simulink model "Conditional_Integrated_Fuzzy_based_Sliding_Mode_Control"  (R2019a)
settings: Solver=FixedStepAuto  StartTime=0.0  StopTime=10  FixedStep=0.001  RelTol=1e-3  EnableMultiTasking=on
InitFcn:
  | %Variable_Entrada
  | Phi_max = 2000;
  | Phi_2  = 20;
  | Phi_1  = 1;
  | Phi_0  = 0;
  | %Variable_Salida
  | U_2= 0.218;
  | U_1 =0.16;
  | U_0  = 0;
  | 
  | %%
  | L =10;
  | Ki =1;
libraries: fuzblock x10
settings Model: Creator=alex_  LastModifiedBy=dell
settings DataIOCC: LimitDataPoints=on  SaveFormat=Array  ReturnWorkspaceOutputs=off
settings OptimizationCC: LifeSpan=inf
settings DebuggingCC: SolverPrmCheckMsg=warning  AllowSymbolicDim=off  SFUnexpectedBacktrackingDiag=warning  SFNoUnconditionalDefaultTransitionDiag=warning  SFExecutionAtInitializationDiag=none  ArithmeticOperatorsInVariantConditions=warning
settings HardwareCC: ProdBitPerPointer=32  ProdBitPerSizeT=32  ProdBitPerPtrDiffT=32  ProdLargestAtomicFloat=None  ProdIntDivRoundTo=Undefined  ProdEndianess=Unspecified  ProdWordSize=32  ProdHWDeviceType=32-bit Generic
settings ModelReferenceCC: PropagateSignalLabelsOutOfModel=off
settings SFSimCC: SimUseLocalCustomCode=off
settings RTWCC: RTWUseLocalCustomCode=off
settings CodeAppCC: StateflowObjectComments=on
settings GRTTargetCC: TargetLangStandard=C89/C90 (ANSI)  GeneratePreprocessorConditionals=Disable all
settings ConfigComp: CovMetricSettings=dw  CovHtmlReporting=on  CovSaveCumulativeToWorkspaceVar=on  CovSaveSingleToWorkspaceVar=on  CovExternalEMLEnable=off  CovSFcnEnable=off
settings SimscapeCC: SimscapeNormalizeSystem=off
settings ConfigurationSet: Description=SimMechanics 2G

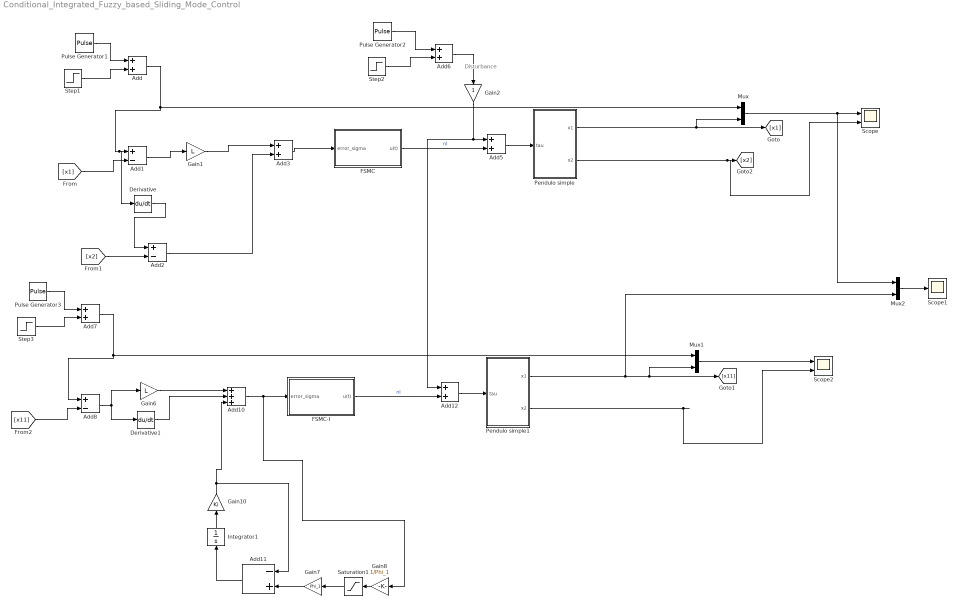
== system Conditional_Integrated_Fuzzy_based_Sliding_Mode_Control ==
  note: Disturbance
  Add{,3,5..7,12} (6 alike) : Sum
  Add1 : Sum  Inputs=+-
  Add10 : Sum  Inputs=+++
  Add11 : Sum  Inputs=-+
  Add2 : Sum  Inputs=+-
  Add8 : Sum  Inputs=+-
  Derivative : Derivative
  Derivative1 : Derivative
  "FSMC " : Subsystem
  FSMC-I : Subsystem
  Gain1 : Gain  Gain=L
  Gain10 : Gain  Gain=Ki
  Gain2 : Gain
  Gain6 : Gain  Gain=L
  Gain7 : Gain  Gain=Phi_1
  Gain8 : Gain  Gain=1/Phi_1
  Integrator1 : Integrator
  Mux : Mux  Inputs=2
  Mux1 : Mux  Inputs=2
  Mux2 : Mux  Inputs=2
  Pendulo simple : Subsystem
  Pendulo simple1 : Subsystem
  Pulse Generator1 : DiscretePulseGenerator  PulseType=Time based  Amplitude=-2  Period=5  PulseWidth=50
  Pulse Generator2 : DiscretePulseGenerator  PulseType=Time based  Amplitude=-0.32  Period=5  PulseWidth=50
  Pulse Generator3 : DiscretePulseGenerator  PulseType=Time based  Amplitude=-2  Period=5  PulseWidth=50
  Saturation1 : Saturate  UpperLimit=1  LowerLimit=-1
  Scope : Scope  NumInputPorts=2
  Scope1 : Scope
  Scope2 : Scope  NumInputPorts=2
  Step1 : Step  Time=0  SampleTime=0
  Step2 : Step  Time=0  After=0.16  SampleTime=0
  Step3 : Step  Time=0  SampleTime=0
  wires:
  Mux/1 -> Mux2/1, Scope/1
  [x2] -> Add2/2
  Pendulo simple/1(x1) -> [x1], Mux/2
  Pendulo simple/2(x2) -> Scope/2, [x2]
  [x1] -> Add1/2
  Add3/1 -> "FSMC "/1(error_sigma)
  Add1/1 -> Gain1/1
  Add2/1 -> Add3/2
  "FSMC "/1(u(t)) -> Add5/2  "nl"
  Gain1/1 -> Add3/1
  Add5/1 -> Pendulo simple/1(tau)
  Pulse Generator2/1 -> Add6/1
  Derivative/1 -> Add2/1
  Step1/1 -> Add/2
  Add/1 -> Mux/1, Derivative/1, Add1/1
  Pulse Generator1/1 -> Add/1
  Step2/1 -> Add6/2
  Pulse Generator3/1 -> Add7/1
  Add6/1 -> Gain2/1
  Add7/1 -> Add8/1, Mux1/1
  Step3/1 -> Add7/2
  Add12/1 -> Pendulo simple1/1(tau)
  Integrator1/1 -> Gain10/1
  Add11/1 -> Integrator1/1
  Gain10/1 -> Add10/3, Add11/1
  Gain7/1 -> Add11/2
  Gain8/1 -> Saturation1/1
  Saturation1/1 -> Gain7/1
  Gain6/1 -> Add10/1
  FSMC-I/1(u(t)) -> Add12/2  "nl"
  Derivative1/1 -> Add10/2
  Add8/1 -> Derivative1/1, Gain6/1
  Add10/1 -> Gain8/1, FSMC-I/1(error_sigma)
  [x11] -> Add8/2
  Pendulo simple1/2(x2) -> Scope2/2
  Pendulo simple1/1(x1) -> Mux2/2, Mux1/2, [x11]
  Mux1/1 -> Scope2/1
  Mux2/1 -> Scope1/1
  Gain2/1 -> Add12/1, Add5/1

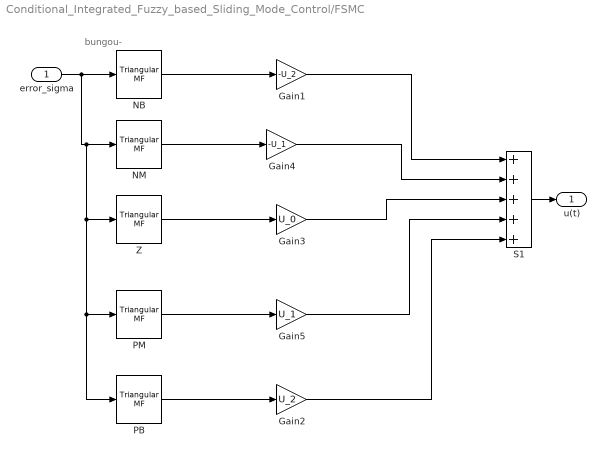
== system Conditional_Integrated_Fuzzy_based_Sliding_Mode_Control/FSMC  ==
  note: bungou-
  error_sigma : Inport
  Gain1 : Gain  Gain=-U_2
  Gain2 : Gain  Gain=U_2
  Gain3 : Gain  Gain=U_0
  Gain4 : Gain  Gain=-U_1
  Gain5 : Gain  Gain=U_1
  NB : fuzblock/Membership  Functions/Triangular MF  a=-Phi_max  b=-Phi_2  c=-Phi_1
      settings: SourceProductName=Fuzzy Logic Toolbox  SourceProductBaseCode=FL
  NM : fuzblock/Membership  Functions/Triangular MF  a=-Phi_2  b=-Phi_1  c=0
      settings: SourceProductName=Fuzzy Logic Toolbox  SourceProductBaseCode=FL
  PB : fuzblock/Membership  Functions/Triangular MF  a=Phi_1  b=Phi_2  c=Phi_max
      settings: SourceProductName=Fuzzy Logic Toolbox  SourceProductBaseCode=FL
  PM : fuzblock/Membership  Functions/Triangular MF  a=0  b=Phi_1  c=Phi_2
      settings: SourceProductName=Fuzzy Logic Toolbox  SourceProductBaseCode=FL
  S1 : Sum  Inputs=+++++  SaturateOnIntegerOverflow=on  InputSameDT=on  OutDataTypeStr=Inherit: Same as first input
  Z : fuzblock/Membership  Functions/Triangular MF  a=-Phi_1  b=0  c=Phi_1
      settings: SourceProductName=Fuzzy Logic Toolbox  SourceProductBaseCode=FL
  u(t) : Outport
  wires:
  NB/1 -> Gain1/1
  Z/1 -> Gain3/1
  PB/1 -> Gain2/1
  PM/1 -> Gain5/1
  Gain1/1 -> S1/1
  Gain4/1 -> S1/2
  Gain3/1 -> S1/3
  Gain2/1 -> S1/5
  Gain5/1 -> S1/4
  error_sigma/1 -> NB/1, NM/1, Z/1, PM/1, PB/1
  S1/1 -> u(t)/1
  NM/1 -> Gain4/1

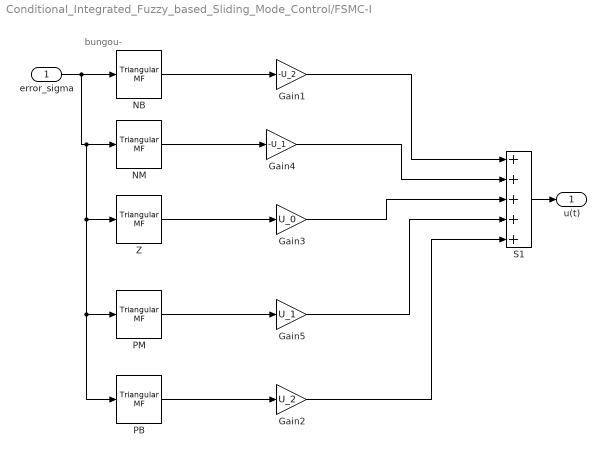
== system Conditional_Integrated_Fuzzy_based_Sliding_Mode_Control/FSMC-I ==
  note: bungou-
  error_sigma : Inport
  Gain1 : Gain  Gain=-U_2
  Gain2 : Gain  Gain=U_2
  Gain3 : Gain  Gain=U_0
  Gain4 : Gain  Gain=-U_1
  Gain5 : Gain  Gain=U_1
  NB : fuzblock/Membership  Functions/Triangular MF  a=-Phi_max  b=-Phi_2  c=-Phi_1
      settings: SourceProductName=Fuzzy Logic Toolbox  SourceProductBaseCode=FL
  NM : fuzblock/Membership  Functions/Triangular MF  a=-Phi_2  b=-Phi_1  c=0
      settings: SourceProductName=Fuzzy Logic Toolbox  SourceProductBaseCode=FL
  PB : fuzblock/Membership  Functions/Triangular MF  a=Phi_1  b=Phi_2  c=Phi_max
      settings: SourceProductName=Fuzzy Logic Toolbox  SourceProductBaseCode=FL
  PM : fuzblock/Membership  Functions/Triangular MF  a=0  b=Phi_1  c=Phi_2
      settings: SourceProductName=Fuzzy Logic Toolbox  SourceProductBaseCode=FL
  S1 : Sum  Inputs=+++++  SaturateOnIntegerOverflow=on  InputSameDT=on  OutDataTypeStr=Inherit: Same as first input
  Z : fuzblock/Membership  Functions/Triangular MF  a=-Phi_1  b=0  c=Phi_1
      settings: SourceProductName=Fuzzy Logic Toolbox  SourceProductBaseCode=FL
  u(t) : Outport
  wires:
  NM/1 -> Gain4/1
  S1/1 -> u(t)/1
  error_sigma/1 -> PB/1, PM/1, Z/1, NM/1, NB/1
  Gain5/1 -> S1/4
  Gain2/1 -> S1/5
  Gain3/1 -> S1/3
  Gain4/1 -> S1/2
  Gain1/1 -> S1/1
  PM/1 -> Gain5/1
  PB/1 -> Gain2/1
  Z/1 -> Gain3/1
  NB/1 -> Gain1/1

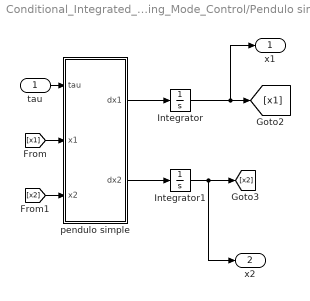
== system Conditional_Integrated_Fuzzy_based_Sliding_Mode_Control/Pendulo simple ==
  tau : Inport
  Integrator : Integrator  InitialCondition=0.1
  Integrator1 : Integrator  InitialCondition=0.1
  pendulo simple : MATLAB Function  TreatAsAtomicUnit=on
  x1 : Outport
  x2 : Outport  Port=2
  wires:
  [x2] -> pendulo simple/3(x2)
  [x1] -> pendulo simple/2(x1)
  tau/1 -> pendulo simple/1(tau)
  pendulo simple/1(dx1) -> Integrator/1
  Integrator/1 -> x1/1, [x1]
  pendulo simple/2(dx2) -> Integrator1/1
  Integrator1/1 -> x2/1, [x2]

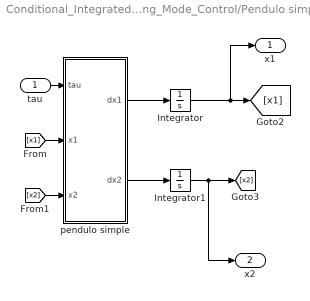
== system Conditional_Integrated_Fuzzy_based_Sliding_Mode_Control/Pendulo simple1 ==
  tau : Inport
  Integrator : Integrator  InitialCondition=0.1
  Integrator1 : Integrator  InitialCondition=0.1
  pendulo simple : MATLAB Function  TreatAsAtomicUnit=on
  x1 : Outport
  x2 : Outport  Port=2
  wires:
  Integrator1/1 -> [x2], x2/1
  pendulo simple/2(dx2) -> Integrator1/1
  Integrator/1 -> [x1], x1/1
  pendulo simple/1(dx1) -> Integrator/1
  tau/1 -> pendulo simple/1(tau)
  [x1] -> pendulo simple/2(x1)
  [x2] -> pendulo simple/3(x2)

== matlab function Conditional_Integrated_Fuzzy_based_Sliding_Mode_Control/Pendulo simple/pendulo simple ==
  data: dx1 output; tau input; x1 input; x2 input; dx2 output
function [dx1,dx2]    = fcn(tau,x1,x2)
%#codegen
J=3.11e-05;
r=100;
g=9.81;
theta1=12.1211973369616;
theta2=0.000243011081164029;
theta3=0.00808832588001993;
theta4=0.00500564359913473;
Jota=J*theta1;
dx1=x2;
dx2=(1/Jota)*(tau-theta2*x2-theta3*tanh(r*x2)-theta4*g*sin(x1));

== matlab function Conditional_Integrated_Fuzzy_based_Sliding_Mode_Control/Pendulo simple1/pendulo simple ==
  data: dx1 output; tau input; x1 input; x2 input; dx2 output
function [dx1,dx2]    = fcn(tau,x1,x2)
%#codegen
J=3.11e-05;
r=100;
g=9.81;
theta1=12.1211973369616;
theta2=0.000243011081164029;
theta3=0.00808832588001993;
theta4=0.00500564359913473;
Jota=J*theta1;
dx1=x2;
dx2=(1/Jota)*(tau-theta2*x2-theta3*tanh(r*x2)-theta4*g*sin(x1));
